simulink model "TwoMotorControllers"  (R2020a)
settings: Solver=ode1  StartTime=0.0  StopTime=Inf  FixedStep=0.001  RelTol=1e-3
PostLoadFcn:
  | , if any(exist('dsrtsu_mdlpostloadfcn', 'file') ~= 0), dsrtsu_mdlpostloadfcn('Execute', bdroot); end,
InitFcn:
  | , if any(exist('rtifpga_mdlclblib', 'file') ~= 0), rtifpga_mdlclblib('Init', bdroot); end,
undefined symbols (not defined in the file): rticanmm_blockfcn, rticanmm_initfcn
libraries: rtimmsu_dsrtlib x2
Description:
  | Standard RTI1401 template.
  | Supported MATLAB version:  R2017b.
settings Model: Tag=RTI1401  DSRTSU_INTERNAL_RTI_VER=560  DSRTSU_INTERNAL_RTI_TYPE=rti1401  RTICANMMDATA=struct('GeneralSetupData',struct('modelroot','C:\Users\harjo\Git\MACFormulaGit\MicroAutobox\microAutoboxModels\MotorTest','generalsettings',struct('filesettings',struct('destfolder',struct('Name','RTICANMM_FILES','Check',1),'buildfolder',struct('Name','.','Check',1),'AbsDestfolder',struct('Name','C:\Users\harjo\Git\MACFormulaGit\MicroAutobox\microAutoboxModels\MotorTest\RTICANMM_FILES'),'AbsBuildfolder',struct('Name','C:\Users\harjo\Git\MACFormulaGit\MicroAutobox\microAutoboxModels\MotorTest'))),'options',struct('addpaths',1,'rmpaths',1,'addtrcexclusion',true,'cannavigator',struct('checkmonitoring',0),'show_usrtrc',0,'use_usrtrc',0,'addpath2usrmk',1),'advanced',struct('options',ones(1,100)),'MPSetup',{{}},'modelname','TwoMotorControllers','blockdata',struct('generalsettings',struct('filesettings',struct('destfolder',struct('Name','.','Check',1),'AbsDestfolder',struct('Name','T:\TOOL_SOURCES\CANnedy\m'),'buildfolder',struct('Name','.','Check',1),'AbsBuildfolder',struct('Name','C:\MATLAB6p5\work'))),'options',struct('addpaths',1,'rmpaths',1,'addpath2usrmk',1),'modelname','rticanmmlib','modelroot','T:\TOOL_SOURCES\CANnedy\m'),'MMType','RTICANMM','block',['TwoMotorControllers/RTICANMM' char(10) 'GeneralSetup'],'RTI',struct('Type','RTI1401','Ver','7.14','Date','02-May-2020'),'version','5.4.737888.359837963','userdata',struct('HostServiceChannelID',{{'Amk'}})))  DSRTSU_INTERNAL_RTIFPGA=160  Creator=Harjot  LastModifiedBy=Harjot
settings OptimizationCC: BlockReduction=off  OptimizeBlockIOStorage=off  BufferReuse=off  GlobalBufferReuse=off  ExpressionFolding=off  LocalBlockOutputs=off  OptimizeDataStoreBuffers=off  BusAssignmentInplaceUpdate=off
settings DebuggingCC: ArithmeticOperatorsInVariantConditions=warning
settings HardwareCC: ProdBitPerPointer=32  ProdBitPerSizeT=32  ProdBitPerPtrDiffT=32  ProdLargestAtomicInteger=Integer  ProdEndianess=BigEndian  ProdWordSize=32  ProdHWDeviceType=Custom Processor->Custom  TargetIntDivRoundTo=Zero  TargetEndianess=BigEndian  TargetHWDeviceType=Custom Processor->Custom
settings SFSimCC: SimUseLocalCustomCode=off  MATLABDynamicMemAlloc=off  CustomCodeUndefinedFunction=UseInterfaceOnly
settings RTWCC: Description=dSPACE DS1401 Hardware Platform  SystemTargetFile=rti1401.tlc  MakeCommand=make_rti  TemplateMakefile=rti1401.tmf  RTWUseLocalCustomCode=off
settings CodeAppCC: StateflowObjectComments=on
settings STFCustomTargetCC: UtilityFuncGeneration=Shared location  ParMdlRefBuildCompliant=on  SystemTargetFile=rti1401.tlc
settings GRTTargetCC: TargetLangStandard=C89/C90 (ANSI)  UtilityFuncGeneration=Shared location  CompOptLevelCompliant=off  ConcurrentExecutionCompliant=off  CombineOutputUpdateFcns=off  MatFileLogging=off  CPPClassGenCompliant=off  UseToolchainInfoCompliant=off
settings ConfigComp: CovMetricSettings=dswe

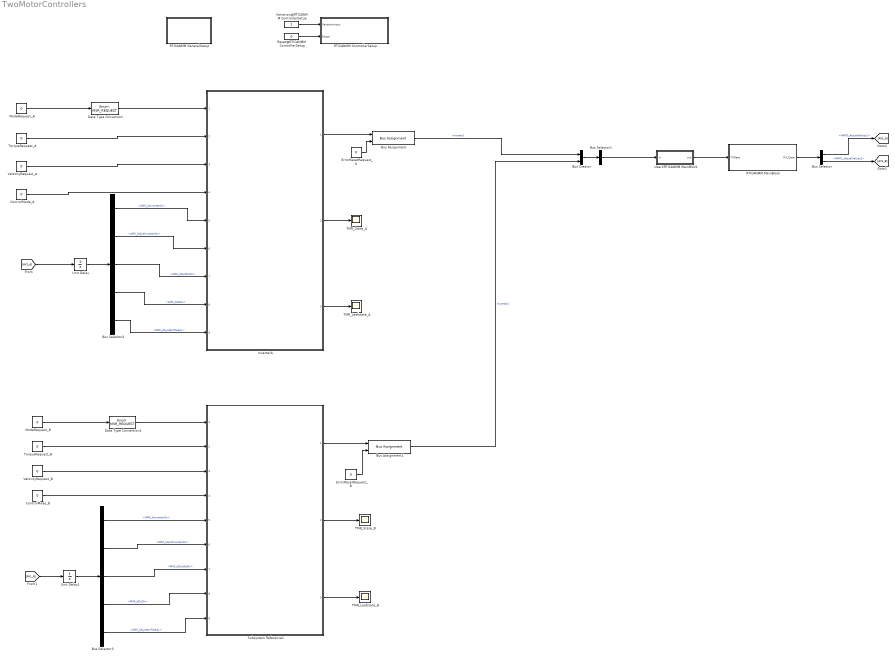
== system TwoMotorControllers ==
  Bus Assignment : BusAssignment  AssignedSignals=AMK_bErrorReset
  Bus Assignment1 : BusAssignment  AssignedSignals=AMK_bErrorReset
  Bus Creator : BusCreator  Inputs=2
  Bus Selector : BusSelector  OutputSignals=AMK0_ActualValues1,AMK1_ActualValues1
  Bus Selector1 : BusSelector  OutputSignals=Inverter1,Inverter2  OutputAsBus=on
  Bus Selector2 : BusSelector  OutputSignals=AMK_bInverterOn,AMK_bQuitInverterOn,AMK_bQuitDcOn,AMK_bDcOn,AMK_bSystemReady
  Bus Selector3 : BusSelector  OutputSignals=AMK_bInverterOn,AMK_bQuitInverterOn,AMK_bQuitDcOn,AMK_bDcOn,AMK_bSystemReady
  ControlMode_A : Constant  Value=0
  ControlMode_B : Constant  Value=0
  Data Type Conversion : DataTypeConversion  OutDataTypeStr=Enum: MSR_REQUEST
  Data Type Conversion1 : DataTypeConversion  OutDataTypeStr=Enum: MSR_REQUEST
  ErrorResetRequest_A : Constant  Value=0  OutDataTypeStr=boolean
  ErrorResetRequest_B : Constant  Value=0  OutDataTypeStr=boolean
  InverterA : Subsystem  ReferencedSubsystem=AMK_Interface
  ModeRequest_A : Constant  Value=0  OutDataTypeStr=uint16
  ModeRequest_B : Constant  Value=0  OutDataTypeStr=uint16
  RTICANMM ControllerSetup : Subsystem  InitFcn=rticanmm_blockfcn('InitFcn', 'CANnedySetup', gcb)  ClipboardFcn=rticanmm_blockfcn('ClipboardFcn', 'CANnedySetup', gcb)  mask(RTICANMM){DSProperties=struct('RTI',struct('Version',uint32(1),'BlockType',struct('isSLSource',uint8(1),'isSLSink',uint8(1),'isHWSource',uint8(0),'isHWSink',uint8(0),'isSetup',uint8(0),'isInline',uint8(1),'isNonInline',uint8(0),'isInterrupt',uint8(0),'isChannelwise',uint8(0)),'IOBoardType','RTICANMM','UnitType','RTICANMM','Identifier','BUSSETUP','DialogType','SL','BlockSet','RTICANMM','SlaveProcessor','CAN')), CANMMProperties=struct('cannedy',struct('data',struct('options',struct('controllername','Amk','controllernameautomatic',[],'loglevel','0','checkrealtime',0,'checkchangebaudrate',0,'sampletime','1.000','CANControllerStatus',0,'NumberofStuffErr',0,'NumberofFormErr',0,'NumberofAckErr',0,'NumberofBit0Err',0,'NumberofsuccrecRX',0,'Numberofsuccsent',0,'NumberofBit1Err',0,'NumberofCRCErr',0,'NumberoflostRX',0,'Busoff',0,'Busload',0,'OperationPending',0,'TxRetryCount',3,'addtrcexclusion',true,'cannavigator',struct('checkmonitoring',0,'checkinternmonitoring',0),'show_usrtrc',0,'use_usrtrc',0,'checkchangebaudrateFD',0,'errorframegeneration',0,'efgenabled',0),'modelroot','C:\Users\harjo\Git\MACFormulaGit\MicroAutobox','generalsettings',struct('setupdata',struct('board',['CAN Type 1'],'boardno',1,'channelno',1,'Type','STD','transceiver','ISO11898-2','busconfig','0x0','feedthrough','false','resistance',struct('r120',1,'roff',0,'r16',1,'r10',0),'baudrate','500','Frequency',[24 36],'samplemode',1,'commChannelTJA1041',6,'config',struct('standard',1,'advanced',0,'register',struct('btr0','0xC0','btr1','0x6F','sp','70','sjw','3','tseg1','15','tseg2','6','brp','0','smpl','0','btr0_36','0x41','btr1_36','0x1E','sp_36','88','sjw_36','1','tseg1_36','14','tseg2_36','1','brp_36','1','smpl_36','0','btr0_64','0x43','btr1_64','0x1C','sp_64','87','sjw_64','1','tseg1_64','12','tseg2_64','1','brp_64','3','smpl_64','0')),'channelcfg',struct('INTENDISABLE','CAN_INT_DISABLE','intenable',0),'SETUPID','RTICANMM_Amk_ID','CONTROLLER_ID','CANMM_CTL_SETUP_Amk','mainblock_includefile','RTICANMM_SETUP_Amk','canfdenable',0,'canfdboardselected',0,'slotno',1,'moduletype','DS4342','baudrateFD','4000','samplePoint','80','samplePointFD','80','termination','TERMINATION_ON'),'filesettings',struct('destfolder',struct('Name','RTICANMM_FILES','Check',1),'buildfolder',struct('Name','.','Check',1))),'advanced',struct('options',ones(1,100)),'partialnetdata',struct('switchedon',0,'format','STD','idmask',['XXXXX XXXXXXXX XXXXXXXX XXXXXXXX'],'idcode','0','idfilter','0','datamaskused',0,'datalength','0','datamask','0x0000000000000000','partialnetworkenable',0)),'blk',['SingleMotorController/RTICANMM' char(10) 'ControllerSetup'],'allgeneratedfiles',{{'C:\Users\harjo\Git\MACFormulaGit\MicroAutobox\microAutoboxModels\MotorTest\RTICANMM_FILES\RTICANMM_SETUP_Amk.c','C:\Users\harjo\Git\MACFormulaGit\MicroAutobox\microAutoboxModels\MotorTest\RTICANMM_FILES\RTICANMM_SETUP_Amk.h','c:\users\harjo\git\macformulagit\microautobox\microautoboxmodels\motortest\rticanmm_files\rticanmm_setup_amk.mexw64'}},'ismp',false,'BlockDataVersion','0.9.0','recreate',0,'CANnedyTag','Amk'),'CANnedynew',0,'CANnedySettings','Amk','GeneratedFiles',{{'C:\Users\harjo\Git\MACFormulaGit\MicroAutobox\microAutoboxModels\MotorTest\RTICANMM_FILES\RTICANMM_SETUP_Amk.c','C:\Users\harjo\Git\MACFormulaGit\MicroAutobox\microAutoboxModels\MotorTest\RTICANMM_FILES\RTICANMM_SETUP_Amk.h','c:\users\harjo\git\macformulagit\microautobox\microautoboxmodels\motortest\rticanmm_files\rticanmm_setup_amk.mexw64'}},'SFCN','RTICANMM_SETUP_Amk.c','HostService',struct('Tags',struct('DATA','RTICANMM_MonitorData','TimeStampGlobal','RTICANMM_MonitoringTimeStamp','TimeStampGlobalEnable','RTICANMM_MonitoringTimeStampEnable','Enable','CANMMMonitor_Amk','TimeStamp','MonitoringTimeStamp_Amk'),'DATA',struct('Length',18),'Info',struct('Desc',{'ID','Service','Data1','Data2','Data3','Data4','Data5','Data6','Data7','Data8','Data9','Data10','Data11','Data12','Data13','Data14','Data15','Data16'}),'Names',struct('TimeStampGlobal','TimeStamp','TimeStampGlobalEnable','TimeStamp_Enable','Enable','Monitoring_Enable','TimeStamp','Monitoring_TimeStamp'),'ChannelID',1)), CANMMType=CANnedySetup, CANMMFolder=C:\Users\harjo\Git\MACFormulaGit\MicroAutobox\microAutoboxModels\MotorTest, CANMMDestFolder=RTICANMM_FILES, CANMMSettings=Amk, CANMMSFcn=RTICANMM_SETUP_Amk, CANMMBoard=DS1401, CANMMBoardNum=1, CANMMChannel=1}
      settings: AttributesFormatString=%<CANMMSettings>: %<CANMMBoard>_B%<CANMMBoardNum>_C%<CANMMChannel>  CopyFcn=rticanmm_blockfcn('CopyFcn', 'CANnedySetup', gcb)  DeleteFcn=rticanmm_blockfcn('DeleteFcn', 'CANnedySetup', gcb)  ModelCloseFcn=rticanmm_blockfcn('ModelCloseFcn', 'CANnedySetup', gcb)  NameChangeFcn=rticanmm_blockfcn('NameChangeFcn', 'CANnedySetup', gcb)  OpenFcn=try, rticanmm_setup_gui('create',gcb); ; catch,errordlg({lasterr, '','Please check your RTI installation.'},['Error: ' upper(bdroot)], 'replace'); end  MoveFcn=rticanmm_blockfcn('MoveFcn', 'CANnedySetup', gcb)
      mask Help: eval('rticanmm_quickstart(''create'', gcb);', 'disp(lasterr);')
      mask Display:
      | disp('RTI CAN\nMultiMessage\nControllerSetup')
      | 
      | port_label('input', 1 , 'Variation')
      | port_label('input', 2 , 'Reset')
  RTICANMM GeneralSetup : Subsystem  InitFcn=rticanmm_initfcn(gcb, 'CANnedySettings')  ClipboardFcn=rticanmm_blockfcn('ClipboardFcn', 'CANnedySettings', gcb)  mask(RTICANMM){DSProperties=struct('RTI',struct('Version',uint32(1),'BlockType',struct('isSLSource',uint8(1),'isSLSink',uint8(1),'isHWSource',uint8(0),'isHWSink',uint8(0),'isSetup',uint8(0),'isInline',uint8(1),'isNonInline',uint8(0),'isInterrupt',uint8(0),'isChannelwise',uint8(0)),'IOBoardType','RTICANMM','UnitType','RTICANMM','Identifier','GENERALSETUP','DialogType','SL','BlockSet','RTICANMM','SlaveProcessor','CAN')), CANMMDestFolder=RTICANMM_FILES, CANMMBuildDir=., CANMMAddPaths=on, CANMMAddpathUserMake=on, CANMMRemovePathOnclose=on, CANMMType=CANnedySettings, CANMMProperties=struct('modelroot','C:\Users\harjo\Git\MACFormulaGit\MicroAutobox\microAutoboxModels\MotorTest','generalsettings',struct('filesettings',struct('destfolder',struct('Name','RTICANMM_FILES','Check',1),'buildfolder',struct('Name','.','Check',1),'AbsDestfolder',struct('Name','C:\Users\harjo\Git\MACFormulaGit\MicroAutobox\microAutoboxModels\MotorTest\RTICANMM_FILES'),'AbsBuildfolder',struct('Name','C:\Users\harjo\Git\MACFormulaGit\MicroAutobox\microAutoboxModels\MotorTest'))),'options',struct('addpaths',1,'rmpaths',1,'addtrcexclusion',true,'cannavigator',struct('checkmonitoring',0),'show_usrtrc',0,'use_usrtrc',0,'addpath2usrmk',1),'advanced',struct('options',ones(1,100)),'MPSetup',{{}},'modelname','TwoMotorControllers','blockdata',struct('generalsettings',struct('filesettings',struct('destfolder',struct('Name','.','Check',1),'AbsDestfolder',struct('Name','T:\TOOL_SOURCES\CANnedy\m'),'buildfolder',struct('Name','.','Check',1),'AbsBuildfolder',struct('Name','C:\MATLAB6p5\work'))),'options',struct('addpaths',1,'rmpaths',1,'addpath2usrmk',1),'modelname','rticanmmlib','modelroot','T:\TOOL_SOURCES\CANnedy\m'),'MMType','RTICANMM','block',['TwoMotorControllers/RTICANMM' char(10) 'GeneralSetup'],'RTI',struct('Type','RTI1401','Ver','7.14','Date','02-May-2020'),'version','5.4.737888.359837963','userdata',struct('HostServiceChannelID',{{'Amk'}}))}
      mask prompts: CANMMDestFolder "Destination Folder for generated Files:"; CANMMBuildDir "Build Directory (*_usr.mk, *_usr.trc)"; CANMMAddPaths "Add Paths automatically"; CANMMAddpathUserMake "Add Paths to UserMake-File"; CANMMRemovePathOnclose "Remove added Path on ModelClose"
      mask init:
      | rticanmm_initfcn(gcb,'CANnedyGeneralSettings')
      settings: CopyFcn=rticanmm_blockfcn('CopyFcn', 'CANnedySettings', gcb)  DeleteFcn=rticanmm_blockfcn('DeleteFcn', 'CANnedySettings', gcb)  ModelCloseFcn=rticanmm_blockfcn('CloseFcn', 'CANnedyGeneralSettings', gcb)  NameChangeFcn=rticanmm_blockfcn('NameChangeFcn', 'CANnedySettings', gcb)  OpenFcn=try, rticanmm_gs_gui('create',gcb), ; catch,errordlg({lasterr, '','Please check your RTI installation.'},['Error: ' upper(bdroot)], 'replace'); end  MoveFcn=rticanmm_blockfcn('MoveFcn', 'CANnedySettings', gcb)
      mask Help: eval('rticanmm_quickstart(''create'', gcb);', 'disp(lasterr);')
      mask Display: disp(sprintf(['RTI CAN\nMultiMessage\nGeneralSetup']))
  RTICANMM MainBlock : Subsystem  InitFcn=rticanmm_blockfcn('InitFcn', 'CANnedy', gcb)  ClipboardFcn=rticanmm_blockfcn('ClipboardFcn', 'CANnedy', gcb)  mask(RTICANMM){DSProperties=struct('RTI',struct('Version',uint32(1),'BlockType',struct('isSLSource',uint8(1),'isSLSink',uint8(1),'isHWSource',uint8(0),'isHWSink',uint8(0),'isSetup',uint8(0),'isInline',uint8(1),'isNonInline',uint8(0),'isInterrupt',uint8(0),'isChannelwise',uint8(0)),'IOBoardType','RTICANMM','UnitType','RTICANMM','Identifier','Mainblock','DialogType','SL','BlockSet','RTICANMM','SlaveProcessor','CAN')), CANMMProperties=struct('RTICANMMVersion','5.4','RTICANMMVersionIntern','5.4.737888.359837963','RTICANMMDate','02-May-2020','Settings','RTICANMM_MAIN_Inverters','UserTracePath','','ModelPath','C:\Users\harjo\Git\MACFormulaGit\MicroAutobox\microAutoboxModels\MotorTest','filesettings',struct('FileName','..\..\..\CAN_Databases\CAN_AMKInverter.dbc','IsRelative',1,'ClusterId',1,'ClusterList',{{'default'}},'destfolder',struct('Name','RTICANMM_FILES','Check',1),'buildfolder',struct('Name','.','Check',1),'onlyfreerawcapture',0,'overlapping2variant',0,'canfdsupport',0,'shortestJ2container',1),'onlyfreerawcapture',0,'Board',['CAN Type 1'],'BoardNum','1','ChannelNum','1','Variation','1','SetupId','Amk','MARK',['842B7A326C18A3163C7749E7722841';'6977FF0AF4BF472FD5A680BD5B0DCB';'8A7174A8B1CB4979025B9E4AAD687D';'AE068A9A32EB922B98A3EA1C91C9E3';'559EEB57A25C395CB78AF64C808C73'],'date','09-Jul-2020','clock',['09.07.2020 22:18:12'],'recreate',0,'RTIVER','RTI1401','j1939',0,'TRC',struct('include',1),'rtsupport',struct('XMLFile','C:\Users\harjo\Git\MACFormulaGit\MicroAutobox\microAutoboxModels\MotorTest\RTICANMM_FILES\RTICANMM_MAIN_Inverters.xml','DBCXML',struct('Path','C:\Users\harjo\Git\MACFormulaGit\MicroAutobox\microAutoboxModels\MotorTest\RTICANMM_FILES\RTICANMM_MAIN_Inverters_dbc.xml','support',1,'Name','CAN_AMKInverter.dbc','Date',['09-Jul-2020 21:47:02'],'Type','standard','DBCSupport','ON'))), CANMMType=CANnedy, CANMMUserTraceMerged=off, CANMMUserTracePath=, CANMMChannelNum=1, CANMMBoardNum=1, CANMMDestFolder=RTICANMM_FILES, CANMMFolder=., CANMMSetupId=Amk, CANMMsave2mat=['842B7A326C18A3163C7749E7722841';'6977FF0AF4BF472FD5A680BD5B0DCB';'8A7174A8B1CB4979025B9E4AAD687D';'AE068A9A32EB922B98A3EA1C91C9E3';'559EEB57A25C395CB78AF64C808C73'], CANMMName=Inverters, CANMMSettings=RTICANMM_MAIN_Inverters, CANMMIntermediateTag=RTICANMM_MAIN_Inverters_intermediate, CANMMsfcnname=RTICANMM_MAIN_Inverters}
      mask init:
      | rticanmm_initfcn(gcb, CANMMType, CANMMsfcnname)
      settings: AttributesFormatString=Amk[Inverters]: DS1401_B1_C1_V1  CopyFcn=rticanmm_blockfcn('CopyFcn', 'CANnedy', gcb)  DeleteFcn=rticanmm_blockfcn('DeleteFcn', 'CANnedy', gcb)  ModelCloseFcn=rticanmm_blockfcn('ModelCloseFcn', 'CANnedy', gcb)  NameChangeFcn=rticanmm_blockfcn('NameChangeFcn', 'CANnedy', gcb)  OpenFcn=try, rticanmm_main_gui('create',gcb); ; catch,errordlg({lasterr, '','Please check your RTI installation.'},['Error: ' upper(bdroot)], 'replace'); end  MoveFcn=rticanmm_blockfcn('MoveFcn', 'CANnedy', gcb)
      mask Help: eval('rticanmm_quickstart(''create'', gcb);', 'disp(lasterr);')
      mask Display:
      | disp(sprintf('RTI CAN\nMultiMessage\nMainBlock'))
      | port_label('input', 1, 'TX Data')
      | port_label('output', 1, 'RX Data')
  Reset@RTICANMM ControllerSetup : Constant  Value=0  OutDataTypeStr=boolean
  Subsystem Reference1 : Subsystem  ReferencedSubsystem=AMK_Interface
  TMR_Leafstate_A : Scope
  TMR_Leafstate_B : Scope
  TMR_State_A : Scope
  TMR_State_B : Scope
  TorqueRequest_A : Constant  Value=0
  TorqueRequest_B : Constant  Value=0
  Unit Delay : UnitDelay  SampleTime=-1  HasFrameUpgradeWarning=on
  Unit Delay1 : UnitDelay  SampleTime=-1  HasFrameUpgradeWarning=on
  User2RTICANMM MainBlock : Subsystem
      mask Display: disp('Mapping\nto RTICANMM')
  Variation@RTICANMM ControllerSetup : Constant  OutDataTypeStr=uint8
  VelocityRequest_A : Constant  Value=0
  VelocityRequest_B : Constant  Value=0
  wires:
  [AV1_A] -> Unit Delay/1
  TorqueRequest_A/1 -> InverterA/2
  VelocityRequest_A/1 -> InverterA/3
  ControlMode_A/1 -> InverterA/4
  Unit Delay/1 -> Bus Selector2/1
  ModeRequest_A/1 -> Data Type Conversion/1
  Data Type Conversion/1 -> InverterA/1
  Variation@RTICANMM ControllerSetup/1 -> RTICANMM ControllerSetup/1(VariationInput)
  Reset@RTICANMM ControllerSetup/1 -> RTICANMM ControllerSetup/2(Reset)
  User2RTICANMM MainBlock/1(out) -> RTICANMM MainBlock/1(TXData)
  RTICANMM MainBlock/1(RX_Data) -> Bus Selector/1
  Bus Selector/1 -> [AV1_A]  "<AMK0_ActualValues1>"
  Bus Selector2/1 -> InverterA/5  "<AMK_bInverterOn>"
  Bus Selector2/2 -> InverterA/6  "<AMK_bQuitInverterOn>"
  Bus Selector2/3 -> InverterA/7  "<AMK_bQuitDcOn>"
  Bus Selector2/4 -> InverterA/8  "<AMK_bDcOn>"
  Bus Selector2/5 -> InverterA/9  "<AMK_bSystemReady>"
  ModeRequest_B/1 -> Data Type Conversion1/1
  ControlMode_B/1 -> Subsystem Reference1/4
  VelocityRequest_B/1 -> Subsystem Reference1/3
  TorqueRequest_B/1 -> Subsystem Reference1/2
  Data Type Conversion1/1 -> Subsystem Reference1/1
  Bus Creator/1 -> Bus Selector1/1
  Bus Selector1/1 -> User2RTICANMM MainBlock/1(in)
  Bus Selector/2 -> [AV1_B]  "<AMK1_ActualValues1>"
  Unit Delay1/1 -> Bus Selector3/1
  [AV1_B] -> Unit Delay1/1
  Bus Selector3/1 -> Subsystem Reference1/5  "<AMK_bInverterOn>"
  Bus Selector3/2 -> Subsystem Reference1/6  "<AMK_bQuitInverterOn>"
  Bus Selector3/3 -> Subsystem Reference1/7  "<AMK_bQuitDcOn>"
  Bus Selector3/4 -> Subsystem Reference1/8  "<AMK_bDcOn>"
  Bus Selector3/5 -> Subsystem Reference1/9  "<AMK_bSystemReady>"
  Bus Assignment/1 -> Bus Creator/1  "Inverter1"
  Bus Assignment1/1 -> Bus Creator/2  "Inverter2"
  InverterA/3 -> TMR_Leafstate_A/1
  InverterA/2 -> TMR_State_A/1
  Subsystem Reference1/2 -> TMR_State_B/1
  Subsystem Reference1/3 -> TMR_Leafstate_B/1
  InverterA/1 -> Bus Assignment/1
  ErrorResetRequest_A/1 -> Bus Assignment/2
  Subsystem Reference1/1 -> Bus Assignment1/1
  ErrorResetRequest_B/1 -> Bus Assignment1/2

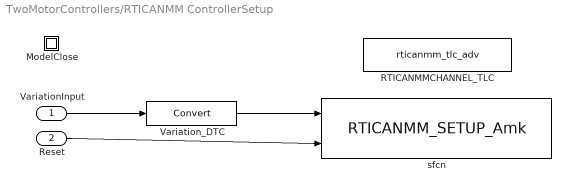
== system TwoMotorControllers/RTICANMM ControllerSetup ==
  VariationInput : Inport
  Reset : Inport  Port=2
  ModelClose : Subsystem  mask(RTICANMMModelClose){}
  RTICANMMCHANNEL_TLC : S-Function  FunctionName=rticanmm_tlc_adv  Parameters=1401,1,1,0,500,11143421  SFunctionDeploymentMode=off  EnableBusSupport=off  mask(RTICANMMCHANNEL_TLC){}
  Variation_DTC : DataTypeConversion  SaturateOnIntegerOverflow=on  RndMeth=Zero
  sfcn : S-Function  InitFcn=rticanmm_initfcn(gcb, 'SFCNs')  FunctionName=RTICANMM_SETUP_Amk  SFunctionDeploymentMode=off  EnableBusSupport=off
      mask init:
      | rticanmm_initfcn(gcb, 'SFCNs')
  wires:
  Reset/1 -> sfcn/2
  VariationInput/1 -> Variation_DTC/1
  Variation_DTC/1 -> sfcn/1

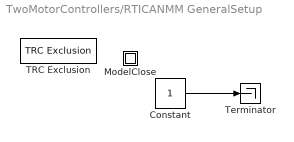
== system TwoMotorControllers/RTICANMM GeneralSetup ==
  Constant : Constant
  ModelClose : Subsystem  mask(RTICANMMModelClose){}
  TRC Exclusion : rtimmsu_dsrtlib/TRC Exclusion
  Terminator : Terminator
  wires:
  Constant/1 -> Terminator/1

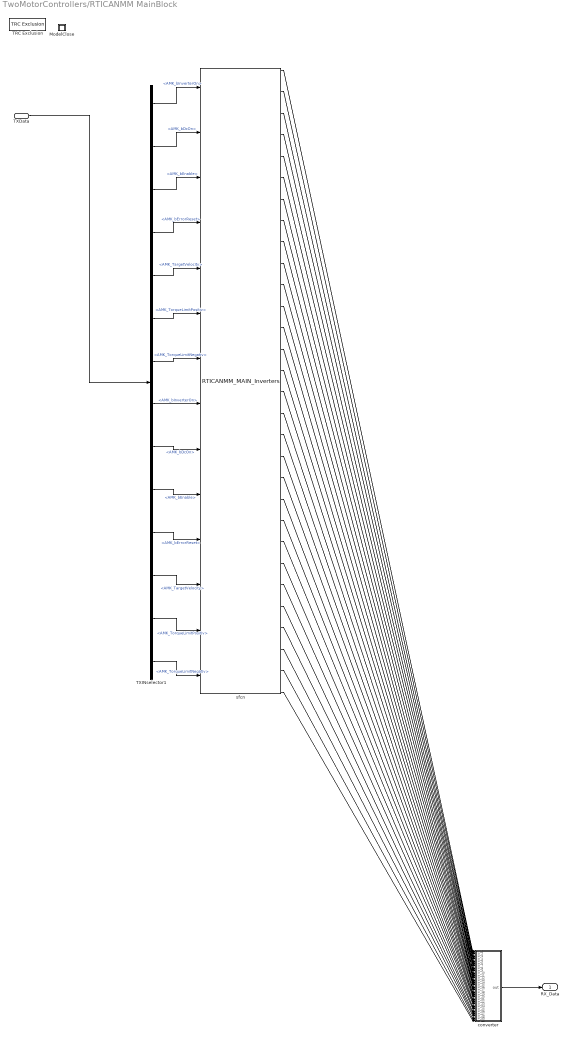
== system TwoMotorControllers/RTICANMM MainBlock ==
  TXData : Inport
  ModelClose : Subsystem  mask(RTICANMMModelClose){}
  TRC Exclusion : rtimmsu_dsrtlib/TRC Exclusion
  TXINselector1 : BusSelector  OutputSignals=AMK0_SetPoints1.AMK_bInverterOn,AMK0_SetPoints1.AMK_bDcOn,AMK0_SetPoints1.AMK_bEnable,AMK0_SetPoints1.AMK_bErrorReset,AMK0_SetPoints1.AMK_TargetVelocity,AMK0_SetPoints1.AMK_TorqueLimitPositiv,AMK0_SetPoints1.AMK_TorqueLimitNegativ,AMK1_SetPoints1.AMK_bInverterOn,AMK1_SetPoints1.AMK_bDcOn,AMK1_SetPoints1.AMK_bEnable,AMK1_SetPoints1.AMK_bErrorReset,AMK1_SetPoints1.AMK_TargetVelocity,AMK1_SetPoints1.AMK_TorqueLimitPositiv,AMK1_SetPoints1.AMK_TorqueLimitNegativ
  converter : Subsystem  mask(CANnedyVector2Bus){}
      mask help: Do not change.
      mask Display: disp('Vector to\nBus')
  sfcn : S-Function  InitFcn=rticanmm_initfcn(gcb, 'SFCNs')  FunctionName=RTICANMM_MAIN_Inverters  SFunctionDeploymentMode=off  EnableBusSupport=off
      mask init:
      | rticanmm_initfcn(gcb, 'SFCNs')
  RX_Data : Outport  VectorParamsAs1DForOutWhenUnconnected=off
  wires:
  TXData/1 -> TXINselector1/1
  TXINselector1/1 -> sfcn/1  "<AMK_bInverterOn>"
  TXINselector1/2 -> sfcn/2  "<AMK_bDcOn>"
  TXINselector1/3 -> sfcn/3  "<AMK_bEnable>"
  TXINselector1/4 -> sfcn/4  "<AMK_bErrorReset>"
  TXINselector1/5 -> sfcn/5  "<AMK_TargetVelocity>"
  TXINselector1/6 -> sfcn/6  "<AMK_TorqueLimitPositiv>"
  TXINselector1/7 -> sfcn/7  "<AMK_TorqueLimitNegativ>"
  TXINselector1/8 -> sfcn/8  "<AMK_bInverterOn>"
  TXINselector1/9 -> sfcn/9  "<AMK_bDcOn>"
  TXINselector1/10 -> sfcn/10  "<AMK_bEnable>"
  TXINselector1/11 -> sfcn/11  "<AMK_bErrorReset>"
  TXINselector1/12 -> sfcn/12  "<AMK_TargetVelocity>"
  TXINselector1/13 -> sfcn/13  "<AMK_TorqueLimitPositiv>"
  TXINselector1/14 -> sfcn/14  "<AMK_TorqueLimitNegativ>"
  converter/1(out) -> RX_Data/1
  sfcn/1 -> converter/1(in_1)
  sfcn/2 -> converter/2(in_2)
  sfcn/3 -> converter/3(in_3)
  sfcn/4 -> converter/4(in_4)
  sfcn/5 -> converter/5(in_5)
  sfcn/6 -> converter/6(in_6)
  sfcn/7 -> converter/7(in_7)
  sfcn/8 -> converter/8(in_8)
  sfcn/9 -> converter/9(in_9)
  sfcn/10 -> converter/10(in_10)
  sfcn/11 -> converter/11(in_11)
  sfcn/12 -> converter/12(in_12)
  sfcn/13 -> converter/13(in_13)
  sfcn/14 -> converter/14(in_14)
  sfcn/15 -> converter/15(in_15)
  sfcn/16 -> converter/16(in_16)
  sfcn/17 -> converter/17(in_17)
  sfcn/18 -> converter/18(in_18)
  sfcn/19 -> converter/19(in_19)
  sfcn/20 -> converter/20(in_20)
  sfcn/21 -> converter/21(in_21)
  sfcn/22 -> converter/22(in_22)
  sfcn/23 -> converter/23(in_23)
  sfcn/24 -> converter/24(in_24)
  sfcn/25 -> converter/25(in_25)
  sfcn/26 -> converter/26(in_26)
  sfcn/27 -> converter/27(in_27)
  sfcn/28 -> converter/28(in_28)
  sfcn/29 -> converter/29(in_29)
  sfcn/30 -> converter/30(in_30)

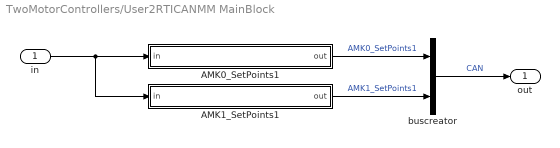
== system TwoMotorControllers/User2RTICANMM MainBlock ==
  in : Inport
  AMK0_SetPoints1 : Subsystem
  AMK1_SetPoints1 : Subsystem
  buscreator : BusCreator  Inputs=2
  out : Outport  VectorParamsAs1DForOutWhenUnconnected=off
  wires:
  AMK0_SetPoints1/1(out) -> buscreator/1  "AMK0_SetPoints1"
  AMK1_SetPoints1/1(out) -> buscreator/2  "AMK1_SetPoints1"
  in/1 -> AMK0_SetPoints1/1(in), AMK1_SetPoints1/1(in)
  buscreator/1 -> out/1  "CAN"

== system TwoMotorControllers/RTICANMM ControllerSetup/ModelClose ==

== system TwoMotorControllers/RTICANMM GeneralSetup/ModelClose ==

== system TwoMotorControllers/RTICANMM MainBlock/ModelClose ==

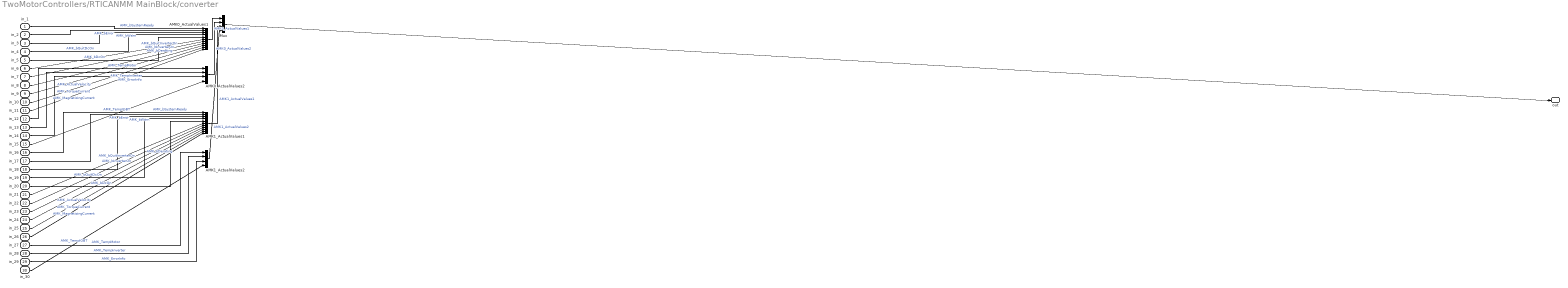
== system TwoMotorControllers/RTICANMM MainBlock/converter ==
  in_1 : Inport
  in_2 : Inport  Port=2
  in_3 : Inport  Port=3
  in_4 : Inport  Port=4
  in_5 : Inport  Port=5
  in_6 : Inport  Port=6
  in_7 : Inport  Port=7
  in_8 : Inport  Port=8
  in_9 : Inport  Port=9
  in_10 : Inport  Port=10
  in_11 : Inport  Port=11
  in_12 : Inport  Port=12
  in_13 : Inport  Port=13
  in_14 : Inport  Port=14
  in_15 : Inport  Port=15
  in_16 : Inport  Port=16
  in_17 : Inport  Port=17
  in_18 : Inport  Port=18
  in_19 : Inport  Port=19
  in_20 : Inport  Port=20
  in_21 : Inport  Port=21
  in_22 : Inport  Port=22
  in_23 : Inport  Port=23
  in_24 : Inport  Port=24
  in_25 : Inport  Port=25
  in_26 : Inport  Port=26
  in_27 : Inport  Port=27
  in_28 : Inport  Port=28
  in_29 : Inport  Port=29
  in_30 : Inport  Port=30
  AMK0_ActualValues1 : BusCreator  Inputs=11
  AMK0_ActualValues2 : BusCreator  Inputs=4
  AMK1_ActualValues1 : BusCreator  Inputs=11
  AMK1_ActualValues2 : BusCreator  Inputs=4
  Mux : BusCreator  Inputs=4
  out : Outport
  wires:
  in_1/1 -> AMK0_ActualValues1/1  "AMK_bSystemReady"
  AMK0_ActualValues1/1 -> Mux/1  "AMK0_ActualValues1"
  in_2/1 -> AMK0_ActualValues1/2  "AMK_bError"
  in_3/1 -> AMK0_ActualValues1/3  "AMK_bWarn"
  in_4/1 -> AMK0_ActualValues1/4  "AMK_bQuitDcOn"
  in_5/1 -> AMK0_ActualValues1/5  "AMK_bDcOn"
  in_6/1 -> AMK0_ActualValues1/6  "AMK_bQuitInverterOn"
  in_7/1 -> AMK0_ActualValues1/7  "AMK_bInverterOn"
  in_8/1 -> AMK0_ActualValues1/8  "AMK_bDerating"
  in_9/1 -> AMK0_ActualValues1/9  "AMK_ActualVelocity"
  in_10/1 -> AMK0_ActualValues1/10  "AMK_TorqueCurrent"
  in_11/1 -> AMK0_ActualValues1/11  "AMK_MagnetizingCurrent"
  in_12/1 -> AMK0_ActualValues2/1  "AMK_TempMotor"
  AMK0_ActualValues2/1 -> Mux/2  "AMK0_ActualValues2"
  in_13/1 -> AMK0_ActualValues2/2  "AMK_TempInverter"
  in_14/1 -> AMK0_ActualValues2/3  "AMK_ErrorInfo"
  in_15/1 -> AMK0_ActualValues2/4  "AMK_TempIGBT"
  in_16/1 -> AMK1_ActualValues1/1  "AMK_bSystemReady"
  AMK1_ActualValues1/1 -> Mux/3  "AMK1_ActualValues1"
  in_17/1 -> AMK1_ActualValues1/2  "AMK_bError"
  in_18/1 -> AMK1_ActualValues1/3  "AMK_bWarn"
  in_19/1 -> AMK1_ActualValues1/4  "AMK_bQuitDcOn"
  in_20/1 -> AMK1_ActualValues1/5  "AMK_bDcOn"
  in_21/1 -> AMK1_ActualValues1/6  "AMK_bQuitInverterOn"
  in_22/1 -> AMK1_ActualValues1/7  "AMK_bInverterOn"
  in_23/1 -> AMK1_ActualValues1/8  "AMK_bDerating"
  in_24/1 -> AMK1_ActualValues1/9  "AMK_ActualVelocity"
  in_25/1 -> AMK1_ActualValues1/10  "AMK_TorqueCurrent"
  in_26/1 -> AMK1_ActualValues1/11  "AMK_MagnetizingCurrent"
  in_27/1 -> AMK1_ActualValues2/1  "AMK_TempMotor"
  AMK1_ActualValues2/1 -> Mux/4  "AMK1_ActualValues2"
  in_28/1 -> AMK1_ActualValues2/2  "AMK_TempInverter"
  in_29/1 -> AMK1_ActualValues2/3  "AMK_ErrorInfo"
  in_30/1 -> AMK1_ActualValues2/4  "AMK_TempIGBT"
  Mux/1 -> out/1

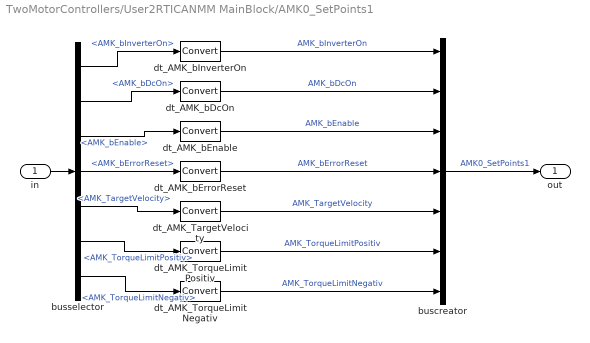
== system TwoMotorControllers/User2RTICANMM MainBlock/AMK0_SetPoints1 ==
  in : Inport
  buscreator : BusCreator  Inputs=7
  busselector : BusSelector  OutputSignals=Inverter1.AMK_bInverterOn,Inverter1.AMK_bDcOn,Inverter1.AMK_bEnable,Inverter1.AMK_bErrorReset,Inverter1.AMK_TargetVelocity,Inverter1.AMK_TorqueLimitPositiv,Inverter1.AMK_TorqueLimitNegativ
  dt_AMK_TargetVelocity : DataTypeConversion  RndMeth=Zero
  dt_AMK_TorqueLimitNegativ : DataTypeConversion  RndMeth=Zero
  dt_AMK_TorqueLimitPositiv : DataTypeConversion  RndMeth=Zero
  dt_AMK_bDcOn : DataTypeConversion  RndMeth=Zero
  dt_AMK_bEnable : DataTypeConversion  RndMeth=Zero
  dt_AMK_bErrorReset : DataTypeConversion  RndMeth=Zero
  dt_AMK_bInverterOn : DataTypeConversion  RndMeth=Zero
  out : Outport
  wires:
  buscreator/1 -> out/1  "AMK0_SetPoints1"
  in/1 -> busselector/1
  busselector/1 -> dt_AMK_bInverterOn/1  "<AMK_bInverterOn>"
  dt_AMK_bInverterOn/1 -> buscreator/1  "AMK_bInverterOn"
  busselector/2 -> dt_AMK_bDcOn/1  "<AMK_bDcOn>"
  dt_AMK_bDcOn/1 -> buscreator/2  "AMK_bDcOn"
  busselector/3 -> dt_AMK_bEnable/1  "<AMK_bEnable>"
  dt_AMK_bEnable/1 -> buscreator/3  "AMK_bEnable"
  busselector/4 -> dt_AMK_bErrorReset/1  "<AMK_bErrorReset>"
  dt_AMK_bErrorReset/1 -> buscreator/4  "AMK_bErrorReset"
  busselector/5 -> dt_AMK_TargetVelocity/1  "<AMK_TargetVelocity>"
  dt_AMK_TargetVelocity/1 -> buscreator/5  "AMK_TargetVelocity"
  busselector/6 -> dt_AMK_TorqueLimitPositiv/1  "<AMK_TorqueLimitPositiv>"
  dt_AMK_TorqueLimitPositiv/1 -> buscreator/6  "AMK_TorqueLimitPositiv"
  busselector/7 -> dt_AMK_TorqueLimitNegativ/1  "<AMK_TorqueLimitNegativ>"
  dt_AMK_TorqueLimitNegativ/1 -> buscreator/7  "AMK_TorqueLimitNegativ"

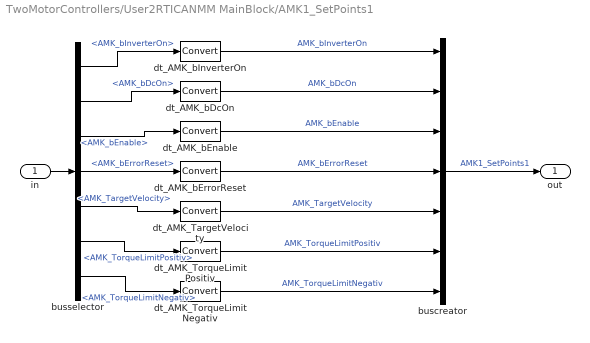
== system TwoMotorControllers/User2RTICANMM MainBlock/AMK1_SetPoints1 ==
  in : Inport
  buscreator : BusCreator  Inputs=7
  busselector : BusSelector  OutputSignals=Inverter2.AMK_bInverterOn,Inverter2.AMK_bDcOn,Inverter2.AMK_bEnable,Inverter2.AMK_bErrorReset,Inverter2.AMK_TargetVelocity,Inverter2.AMK_TorqueLimitPositiv,Inverter2.AMK_TorqueLimitNegativ
  dt_AMK_TargetVelocity : DataTypeConversion  RndMeth=Zero
  dt_AMK_TorqueLimitNegativ : DataTypeConversion  RndMeth=Zero
  dt_AMK_TorqueLimitPositiv : DataTypeConversion  RndMeth=Zero
  dt_AMK_bDcOn : DataTypeConversion  RndMeth=Zero
  dt_AMK_bEnable : DataTypeConversion  RndMeth=Zero
  dt_AMK_bErrorReset : DataTypeConversion  RndMeth=Zero
  dt_AMK_bInverterOn : DataTypeConversion  RndMeth=Zero
  out : Outport
  wires:
  buscreator/1 -> out/1  "AMK1_SetPoints1"
  in/1 -> busselector/1
  busselector/1 -> dt_AMK_bInverterOn/1  "<AMK_bInverterOn>"
  dt_AMK_bInverterOn/1 -> buscreator/1  "AMK_bInverterOn"
  busselector/2 -> dt_AMK_bDcOn/1  "<AMK_bDcOn>"
  dt_AMK_bDcOn/1 -> buscreator/2  "AMK_bDcOn"
  busselector/3 -> dt_AMK_bEnable/1  "<AMK_bEnable>"
  dt_AMK_bEnable/1 -> buscreator/3  "AMK_bEnable"
  busselector/4 -> dt_AMK_bErrorReset/1  "<AMK_bErrorReset>"
  dt_AMK_bErrorReset/1 -> buscreator/4  "AMK_bErrorReset"
  busselector/5 -> dt_AMK_TargetVelocity/1  "<AMK_TargetVelocity>"
  dt_AMK_TargetVelocity/1 -> buscreator/5  "AMK_TargetVelocity"
  busselector/6 -> dt_AMK_TorqueLimitPositiv/1  "<AMK_TorqueLimitPositiv>"
  dt_AMK_TorqueLimitPositiv/1 -> buscreator/6  "AMK_TorqueLimitPositiv"
  busselector/7 -> dt_AMK_TorqueLimitNegativ/1  "<AMK_TorqueLimitNegativ>"
  dt_AMK_TorqueLimitNegativ/1 -> buscreator/7  "AMK_TorqueLimitNegativ"
